simulink subsystem "AeroPropRefFranc"  (R2024b)
settings: Solver=VariableStepAuto  StartTime=0.0  StopTime=10.0  RelTol=1e-3
undefined symbols (not defined in the file or in its folder): ess, Force_b, Fprop_r, geom, H_b, Hdot_b, Moment_b, mot, mot2, mot3, mot4, Mprop_r, propel, propel2, propel3, propel4, pxf_diagram_options, SimIn, SimPar, tc, tc2, tc3, tc4
libraries: simulink x8, slpidlib x4, starslibAxisTransformations x2, libAxisTransformations x2
(part 5 of 10)

== system AeroPropRefFranc/Propulsion and Aerodynamic Forces and Moments/S-Function/Battery Model/powerplant/propel2/plant/parameter_out ==
  inport-propel2_plant_speed_simu : Inport
  inport-propel2_plant_pwr_in_simu : Inport  Port=2
  inport-propel2_plant_pwr_out_simu : Inport  Port=3
  inport-propel2_plant_thrust_simu : Inport  Port=4
  Toworkspace-propel2_plant_pwr_in_simu : ToWorkspace  VariableName=propel2_plant_pwr_in_simu  SampleTime=pxf_diagram_options.workspace_sample_time
      settings: Decimation=pxf_diagram_options.decimation
  Toworkspace-propel2_plant_pwr_out_simu : ToWorkspace  VariableName=propel2_plant_pwr_out_simu  SampleTime=pxf_diagram_options.workspace_sample_time
      settings: Decimation=pxf_diagram_options.decimation
  Toworkspace-propel2_plant_speed_simu : ToWorkspace  VariableName=propel2_plant_speed_simu  SampleTime=pxf_diagram_options.workspace_sample_time
      settings: Decimation=pxf_diagram_options.decimation
  Toworkspace-propel2_plant_thrust_simu : ToWorkspace  VariableName=propel2_plant_thrust_simu  SampleTime=pxf_diagram_options.workspace_sample_time
      settings: Decimation=pxf_diagram_options.decimation
  create_system_info_bus : BusCreator  Inputs=1
  outport-system_info_bus : Outport
  wires:
  inport-propel2_plant_thrust_simu/1 -> Toworkspace-propel2_plant_thrust_simu/1
  inport-propel2_plant_pwr_out_simu/1 -> Toworkspace-propel2_plant_pwr_out_simu/1
  inport-propel2_plant_pwr_in_simu/1 -> Toworkspace-propel2_plant_pwr_in_simu/1
  inport-propel2_plant_speed_simu/1 -> Toworkspace-propel2_plant_speed_simu/1, create_system_info_bus/1  "propel2_plant_speed_simu"
  create_system_info_bus/1 -> outport-system_info_bus/1

== system AeroPropRefFranc/Propulsion and Aerodynamic Forces and Moments/S-Function/Battery Model/powerplant/propel2/plant/parameter_selection ==
  inport-main_info_bus-1 : Inport
  select_main_info_bus : BusSelector  OutputSignals=env_info_bus.env_plant_density_simu,apa_info_bus.powerplant_info_bus.tc.tc_plant_inertia_out_simu,apa_info_bus.apa_plant_info_bus.apa_plant_info_bus.forceeq_bus.eqnmotion_plant_linvel_simu
  outport-env_plant_density_simu-1 : Outport
  outport-tc_plant_inertia_out_simu-2 : Outport  Port=2
  outport-eqnmotion_plant_linvel_simu-3 : Outport  Port=3
  wires:
  select_main_info_bus/3 -> outport-eqnmotion_plant_linvel_simu-3/1  "<eqnmotion_plant_linvel_simu>"
  select_main_info_bus/2 -> outport-tc_plant_inertia_out_simu-2/1  "<tc_plant_inertia_out_simu>"
  select_main_info_bus/1 -> outport-env_plant_density_simu-1/1  "<env_plant_density_simu>"
  inport-main_info_bus-1/1 -> select_main_info_bus/1

== system AeroPropRefFranc/Propulsion and Aerodynamic Forces and Moments/S-Function/Battery Model/powerplant/propel2/plant/propel2_plant_uas ==
  note: rev/s
  note: rad/s
  env_plant_density_simu : Inport
  tc_plant_inertia_out_simu : Inport  Port=2
  eqnmotion_plant_linvel_simu : Inport  Port=3
  tc_plant_trq_out_simu : Inport  Port=4
  flow-in : Inport  Port=5
  Gain : Gain  Gain=propel2.plant.init.thrustdir
  Gain1 : Gain  Gain=2*pi
  Gain2 : Gain
  Gain3 : Gain
  Mux : Mux  Inputs=2
  Propeller Power : Subsystem
  Propeller_CP : Subsystem
  Propeller_Torque : Subsystem
  Terminator : Terminator
  Thrust_Generated : Subsystem
  Total_Moment : Subsystem
  propel_plant_speed_simu : Outport  VectorParamsAs1DForOutWhenUnconnected=off
  propel_plant_pwr_in_simu : Outport  Port=2  VectorParamsAs1DForOutWhenUnconnected=off
  propel_plant_pwr_out_simu : Outport  Port=3  VectorParamsAs1DForOutWhenUnconnected=off
  propel_plant_thrust_simu : Outport  Port=4  VectorParamsAs1DForOutWhenUnconnected=off
  propel_plant_effort : Outport  Port=5  VectorParamsAs1DForOutWhenUnconnected=off
  propel_plant_speed_out_simu : Outport  Port=6  VectorParamsAs1DForOutWhenUnconnected=off
  wires:
  Thrust_Generated/1(propel_plant_thrust_simu) -> propel_plant_thrust_simu/1, Gain/1, Total_Moment/1(propel_plant_thrust_simu), Propeller Power/3(propel_plant_thrust_simu)  "propel_plant_thrust_simu"
  Propeller_Torque/1(propel_plant_rps_simu) -> Thrust_Generated/2(propel_plant_speed_simu), Propeller_CP/1(propel_plant_rps_simu), Gain1/1, Propeller Power/4(propel_plant_rps_simu)
  Propeller_CP/1(propel_plant_CP_simu) -> Propeller_Torque/2(propel_plant_CP_simu), Propeller Power/2(propel_plant_CP_simu)
  Thrust_Generated/2(propel_plant_CT_simu) -> Propeller Power/1(propel_plant_CT_simu)
  env_plant_density_simu/1 -> Propeller_Torque/1(env_plant_density_simu), Thrust_Generated/1(env_plant_density_simu)
  tc_plant_trq_out_simu/1 -> Propeller_Torque/3(tc_plant_trq_out_simu)
  tc_plant_inertia_out_simu/1 -> Propeller_Torque/4(tc_plant_inertia_out_simu)
  Total_Moment/1(accmoment_plant_totmoment_simu) -> Mux/2  "effort_plant_angleffort_simu"
  Propeller_Torque/2(propel_plant_restq_simu) -> Total_Moment/2(propel_plant_restq_simu)
  Gain/1 -> Mux/1  "effort_plant_longeffort_simu"
  Mux/1 -> propel_plant_effort/1  "propel_plant_effort"
  eqnmotion_plant_linvel_simu/1 -> Propeller Power/5(eqnmotion_plant_linvel_simu)
  Gain1/1 -> Gain3/1, Gain2/1
  Propeller Power/2(propel_plant_pwr_out_simu) -> propel_plant_pwr_out_simu/1  "propel_plant_pwr_out_simu"
  Propeller Power/1(propel_plant_pwr_in_simu) -> propel_plant_pwr_in_simu/1  "propel_plant_pwr_in_simu"
  Gain2/1 -> propel_plant_speed_out_simu/1  "propel_plant_speed_out_simu"
  Gain3/1 -> propel_plant_speed_simu/1  "propel_plant_speed_simu"
  flow-in/1 -> Terminator/1

== system AeroPropRefFranc/Propulsion and Aerodynamic Forces and Moments/S-Function/Battery Model/powerplant/propel3/plant/parameter_out ==
  inport-propel3_plant_speed_simu : Inport
  inport-propel3_plant_pwr_in_simu : Inport  Port=2
  inport-propel3_plant_pwr_out_simu : Inport  Port=3
  inport-propel3_plant_thrust_simu : Inport  Port=4
  Toworkspace-propel3_plant_pwr_in_simu : ToWorkspace  VariableName=propel3_plant_pwr_in_simu  SampleTime=pxf_diagram_options.workspace_sample_time
      settings: Decimation=pxf_diagram_options.decimation
  Toworkspace-propel3_plant_pwr_out_simu : ToWorkspace  VariableName=propel3_plant_pwr_out_simu  SampleTime=pxf_diagram_options.workspace_sample_time
      settings: Decimation=pxf_diagram_options.decimation
  Toworkspace-propel3_plant_speed_simu : ToWorkspace  VariableName=propel3_plant_speed_simu  SampleTime=pxf_diagram_options.workspace_sample_time
      settings: Decimation=pxf_diagram_options.decimation
  Toworkspace-propel3_plant_thrust_simu : ToWorkspace  VariableName=propel3_plant_thrust_simu  SampleTime=pxf_diagram_options.workspace_sample_time
      settings: Decimation=pxf_diagram_options.decimation
  create_system_info_bus : BusCreator  Inputs=1
  outport-system_info_bus : Outport
  wires:
  inport-propel3_plant_thrust_simu/1 -> Toworkspace-propel3_plant_thrust_simu/1
  inport-propel3_plant_pwr_out_simu/1 -> Toworkspace-propel3_plant_pwr_out_simu/1
  inport-propel3_plant_pwr_in_simu/1 -> Toworkspace-propel3_plant_pwr_in_simu/1
  inport-propel3_plant_speed_simu/1 -> Toworkspace-propel3_plant_speed_simu/1, create_system_info_bus/1  "propel3_plant_speed_simu"
  create_system_info_bus/1 -> outport-system_info_bus/1

== system AeroPropRefFranc/Propulsion and Aerodynamic Forces and Moments/S-Function/Battery Model/powerplant/propel3/plant/parameter_selection ==
  inport-main_info_bus-1 : Inport
  select_main_info_bus : BusSelector  OutputSignals=env_info_bus.env_plant_density_simu,apa_info_bus.powerplant_info_bus.tc.tc_plant_inertia_out_simu,apa_info_bus.apa_plant_info_bus.apa_plant_info_bus.forceeq_bus.eqnmotion_plant_linvel_simu
  outport-env_plant_density_simu-1 : Outport
  outport-tc_plant_inertia_out_simu-2 : Outport  Port=2
  outport-eqnmotion_plant_linvel_simu-3 : Outport  Port=3
  wires:
  select_main_info_bus/3 -> outport-eqnmotion_plant_linvel_simu-3/1  "<eqnmotion_plant_linvel_simu>"
  select_main_info_bus/2 -> outport-tc_plant_inertia_out_simu-2/1  "<tc_plant_inertia_out_simu>"
  select_main_info_bus/1 -> outport-env_plant_density_simu-1/1  "<env_plant_density_simu>"
  inport-main_info_bus-1/1 -> select_main_info_bus/1

== system AeroPropRefFranc/Propulsion and Aerodynamic Forces and Moments/S-Function/Battery Model/powerplant/propel3/plant/propel3_plant_uas ==
  note: rev/s
  note: rad/s
  env_plant_density_simu : Inport
  tc_plant_inertia_out_simu : Inport  Port=2
  eqnmotion_plant_linvel_simu : Inport  Port=3
  tc_plant_trq_out_simu : Inport  Port=4
  flow-in : Inport  Port=5
  Gain : Gain  Gain=propel3.plant.init.thrustdir
  Gain1 : Gain  Gain=2*pi
  Gain2 : Gain
  Gain3 : Gain
  Mux : Mux  Inputs=2
  Propeller Power : Subsystem
  Propeller_CP : Subsystem
  Propeller_Torque : Subsystem
  Terminator : Terminator
  Thrust_Generated : Subsystem
  Total_Moment : Subsystem
  propel_plant_speed_simu : Outport  VectorParamsAs1DForOutWhenUnconnected=off
  propel_plant_pwr_in_simu : Outport  Port=2  VectorParamsAs1DForOutWhenUnconnected=off
  propel_plant_pwr_out_simu : Outport  Port=3  VectorParamsAs1DForOutWhenUnconnected=off
  propel_plant_thrust_simu : Outport  Port=4  VectorParamsAs1DForOutWhenUnconnected=off
  propel_plant_effort : Outport  Port=5  VectorParamsAs1DForOutWhenUnconnected=off
  propel_plant_speed_out_simu : Outport  Port=6  VectorParamsAs1DForOutWhenUnconnected=off
  wires:
  Thrust_Generated/1(propel_plant_thrust_simu) -> propel_plant_thrust_simu/1, Gain/1, Total_Moment/1(propel_plant_thrust_simu), Propeller Power/3(propel_plant_thrust_simu)  "propel_plant_thrust_simu"
  Propeller_Torque/1(propel_plant_rps_simu) -> Thrust_Generated/2(propel_plant_speed_simu), Propeller_CP/1(propel_plant_rps_simu), Gain1/1, Propeller Power/4(propel_plant_rps_simu)
  Propeller_CP/1(propel_plant_CP_simu) -> Propeller_Torque/2(propel_plant_CP_simu), Propeller Power/2(propel_plant_CP_simu)
  Thrust_Generated/2(propel_plant_CT_simu) -> Propeller Power/1(propel_plant_CT_simu)
  env_plant_density_simu/1 -> Propeller_Torque/1(env_plant_density_simu), Thrust_Generated/1(env_plant_density_simu)
  tc_plant_trq_out_simu/1 -> Propeller_Torque/3(tc_plant_trq_out_simu)
  tc_plant_inertia_out_simu/1 -> Propeller_Torque/4(tc_plant_inertia_out_simu)
  Total_Moment/1(accmoment_plant_totmoment_simu) -> Mux/2  "effort_plant_angleffort_simu"
  Propeller_Torque/2(propel_plant_restq_simu) -> Total_Moment/2(propel_plant_restq_simu)
  Gain/1 -> Mux/1  "effort_plant_longeffort_simu"
  Mux/1 -> propel_plant_effort/1  "propel_plant_effort"
  eqnmotion_plant_linvel_simu/1 -> Propeller Power/5(eqnmotion_plant_linvel_simu)
  Gain1/1 -> Gain3/1, Gain2/1
  Propeller Power/2(propel_plant_pwr_out_simu) -> propel_plant_pwr_out_simu/1  "propel_plant_pwr_out_simu"
  Propeller Power/1(propel_plant_pwr_in_simu) -> propel_plant_pwr_in_simu/1  "propel_plant_pwr_in_simu"
  Gain2/1 -> propel_plant_speed_out_simu/1  "propel_plant_speed_out_simu"
  Gain3/1 -> propel_plant_speed_simu/1  "propel_plant_speed_simu"
  flow-in/1 -> Terminator/1

== system AeroPropRefFranc/Propulsion and Aerodynamic Forces and Moments/S-Function/Battery Model/powerplant/propel4/plant/parameter_out ==
  inport-propel4_plant_speed_simu : Inport
  inport-propel4_plant_pwr_in_simu : Inport  Port=2
  inport-propel4_plant_pwr_out_simu : Inport  Port=3
  inport-propel4_plant_thrust_simu : Inport  Port=4
  Toworkspace-propel4_plant_pwr_in_simu : ToWorkspace  VariableName=propel4_plant_pwr_in_simu  SampleTime=pxf_diagram_options.workspace_sample_time
      settings: Decimation=pxf_diagram_options.decimation
  Toworkspace-propel4_plant_pwr_out_simu : ToWorkspace  VariableName=propel4_plant_pwr_out_simu  SampleTime=pxf_diagram_options.workspace_sample_time
      settings: Decimation=pxf_diagram_options.decimation
  Toworkspace-propel4_plant_speed_simu : ToWorkspace  VariableName=propel4_plant_speed_simu  SampleTime=pxf_diagram_options.workspace_sample_time
      settings: Decimation=pxf_diagram_options.decimation
  Toworkspace-propel4_plant_thrust_simu : ToWorkspace  VariableName=propel4_plant_thrust_simu  SampleTime=pxf_diagram_options.workspace_sample_time
      settings: Decimation=pxf_diagram_options.decimation
  create_system_info_bus : BusCreator  Inputs=1
  outport-system_info_bus : Outport
  wires:
  inport-propel4_plant_thrust_simu/1 -> Toworkspace-propel4_plant_thrust_simu/1
  inport-propel4_plant_pwr_out_simu/1 -> Toworkspace-propel4_plant_pwr_out_simu/1
  inport-propel4_plant_pwr_in_simu/1 -> Toworkspace-propel4_plant_pwr_in_simu/1
  inport-propel4_plant_speed_simu/1 -> Toworkspace-propel4_plant_speed_simu/1, create_system_info_bus/1  "propel4_plant_speed_simu"
  create_system_info_bus/1 -> outport-system_info_bus/1

== system AeroPropRefFranc/Propulsion and Aerodynamic Forces and Moments/S-Function/Battery Model/powerplant/propel4/plant/parameter_selection ==
  inport-main_info_bus-1 : Inport
  select_main_info_bus : BusSelector  OutputSignals=env_info_bus.env_plant_density_simu,apa_info_bus.powerplant_info_bus.tc.tc_plant_inertia_out_simu,apa_info_bus.apa_plant_info_bus.apa_plant_info_bus.forceeq_bus.eqnmotion_plant_linvel_simu
  outport-env_plant_density_simu-1 : Outport
  outport-tc_plant_inertia_out_simu-2 : Outport  Port=2
  outport-eqnmotion_plant_linvel_simu-3 : Outport  Port=3
  wires:
  select_main_info_bus/3 -> outport-eqnmotion_plant_linvel_simu-3/1  "<eqnmotion_plant_linvel_simu>"
  select_main_info_bus/2 -> outport-tc_plant_inertia_out_simu-2/1  "<tc_plant_inertia_out_simu>"
  select_main_info_bus/1 -> outport-env_plant_density_simu-1/1  "<env_plant_density_simu>"
  inport-main_info_bus-1/1 -> select_main_info_bus/1

== system AeroPropRefFranc/Propulsion and Aerodynamic Forces and Moments/S-Function/Battery Model/powerplant/propel4/plant/propel4_plant_uas ==
  note: rev/s
  note: rad/s
  env_plant_density_simu : Inport
  tc_plant_inertia_out_simu : Inport  Port=2
  eqnmotion_plant_linvel_simu : Inport  Port=3
  tc_plant_trq_out_simu : Inport  Port=4
  flow-in : Inport  Port=5
  Gain : Gain  Gain=propel4.plant.init.thrustdir
  Gain1 : Gain  Gain=2*pi
  Gain2 : Gain
  Gain3 : Gain
  Mux : Mux  Inputs=2
  Propeller Power : Subsystem
  Propeller_CP : Subsystem
  Propeller_Torque : Subsystem
  Terminator : Terminator
  Thrust_Generated : Subsystem
  Total_Moment : Subsystem
  propel_plant_speed_simu : Outport  VectorParamsAs1DForOutWhenUnconnected=off
  propel_plant_pwr_in_simu : Outport  Port=2  VectorParamsAs1DForOutWhenUnconnected=off
  propel_plant_pwr_out_simu : Outport  Port=3  VectorParamsAs1DForOutWhenUnconnected=off
  propel_plant_thrust_simu : Outport  Port=4  VectorParamsAs1DForOutWhenUnconnected=off
  propel_plant_effort : Outport  Port=5  VectorParamsAs1DForOutWhenUnconnected=off
  propel_plant_speed_out_simu : Outport  Port=6  VectorParamsAs1DForOutWhenUnconnected=off
  wires:
  Thrust_Generated/1(propel_plant_thrust_simu) -> propel_plant_thrust_simu/1, Gain/1, Total_Moment/1(propel_plant_thrust_simu), Propeller Power/3(propel_plant_thrust_simu)  "propel_plant_thrust_simu"
  Propeller_Torque/1(propel_plant_rps_simu) -> Thrust_Generated/2(propel_plant_speed_simu), Propeller_CP/1(propel_plant_rps_simu), Gain1/1, Propeller Power/4(propel_plant_rps_simu)
  Propeller_CP/1(propel_plant_CP_simu) -> Propeller_Torque/2(propel_plant_CP_simu), Propeller Power/2(propel_plant_CP_simu)
  Thrust_Generated/2(propel_plant_CT_simu) -> Propeller Power/1(propel_plant_CT_simu)
  env_plant_density_simu/1 -> Propeller_Torque/1(env_plant_density_simu), Thrust_Generated/1(env_plant_density_simu)
  tc_plant_trq_out_simu/1 -> Propeller_Torque/3(tc_plant_trq_out_simu)
  tc_plant_inertia_out_simu/1 -> Propeller_Torque/4(tc_plant_inertia_out_simu)
  Total_Moment/1(accmoment_plant_totmoment_simu) -> Mux/2  "effort_plant_angleffort_simu"
  Propeller_Torque/2(propel_plant_restq_simu) -> Total_Moment/2(propel_plant_restq_simu)
  Gain/1 -> Mux/1  "effort_plant_longeffort_simu"
  Mux/1 -> propel_plant_effort/1  "propel_plant_effort"
  eqnmotion_plant_linvel_simu/1 -> Propeller Power/5(eqnmotion_plant_linvel_simu)
  Gain1/1 -> Gain3/1, Gain2/1
  Propeller Power/2(propel_plant_pwr_out_simu) -> propel_plant_pwr_out_simu/1  "propel_plant_pwr_out_simu"
  Propeller Power/1(propel_plant_pwr_in_simu) -> propel_plant_pwr_in_simu/1  "propel_plant_pwr_in_simu"
  Gain2/1 -> propel_plant_speed_out_simu/1  "propel_plant_speed_out_simu"
  Gain3/1 -> propel_plant_speed_simu/1  "propel_plant_speed_simu"
  flow-in/1 -> Terminator/1

== system AeroPropRefFranc/Propulsion and Aerodynamic Forces and Moments/S-Function/Battery Model/powerplant/tc/plant/parameter_out ==
  inport-tc_plant_trq_in_simu : Inport
  inport-tc_plant_trq_out_simu : Inport  Port=2
  inport-tc_plant_spd_in_simu : Inport  Port=3
  inport-tc_plant_spd_out_simu : Inport  Port=4
  inport-tc_plant_inertia_in_simu : Inport  Port=5
  inport-tc_plant_inertia_out_simu : Inport  Port=6
  Toworkspace-tc_plant_inertia_in_simu : ToWorkspace  VariableName=tc_plant_inertia_in_simu  SampleTime=pxf_diagram_options.workspace_sample_time
      settings: Decimation=pxf_diagram_options.decimation
  Toworkspace-tc_plant_inertia_out_simu : ToWorkspace  VariableName=tc_plant_inertia_out_simu  SampleTime=pxf_diagram_options.workspace_sample_time
      settings: Decimation=pxf_diagram_options.decimation
  Toworkspace-tc_plant_spd_in_simu : ToWorkspace  VariableName=tc_plant_spd_in_simu  SampleTime=pxf_diagram_options.workspace_sample_time
      settings: Decimation=pxf_diagram_options.decimation
  Toworkspace-tc_plant_spd_out_simu : ToWorkspace  VariableName=tc_plant_spd_out_simu  SampleTime=pxf_diagram_options.workspace_sample_time
      settings: Decimation=pxf_diagram_options.decimation
  Toworkspace-tc_plant_trq_in_simu : ToWorkspace  VariableName=tc_plant_trq_in_simu  SampleTime=pxf_diagram_options.workspace_sample_time
      settings: Decimation=pxf_diagram_options.decimation
  Toworkspace-tc_plant_trq_out_simu : ToWorkspace  VariableName=tc_plant_trq_out_simu  SampleTime=pxf_diagram_options.workspace_sample_time
      settings: Decimation=pxf_diagram_options.decimation
  create_system_info_bus : BusCreator  Inputs=2
  outport-system_info_bus : Outport
  wires:
  inport-tc_plant_inertia_out_simu/1 -> Toworkspace-tc_plant_inertia_out_simu/1, create_system_info_bus/2  "tc_plant_inertia_out_simu"
  inport-tc_plant_inertia_in_simu/1 -> Toworkspace-tc_plant_inertia_in_simu/1
  inport-tc_plant_spd_out_simu/1 -> Toworkspace-tc_plant_spd_out_simu/1
  inport-tc_plant_spd_in_simu/1 -> Toworkspace-tc_plant_spd_in_simu/1, create_system_info_bus/1  "tc_plant_spd_in_simu"
  inport-tc_plant_trq_out_simu/1 -> Toworkspace-tc_plant_trq_out_simu/1
  inport-tc_plant_trq_in_simu/1 -> Toworkspace-tc_plant_trq_in_simu/1
  create_system_info_bus/1 -> outport-system_info_bus/1

== system AeroPropRefFranc/Propulsion and Aerodynamic Forces and Moments/S-Function/Battery Model/powerplant/tc/plant/parameter_selection ==

== system AeroPropRefFranc/Propulsion and Aerodynamic Forces and Moments/S-Function/Battery Model/powerplant/tc/plant/tc_plant_map_trqloss_funTW ==
  tc_trq_in tc_inertia_in : Inport
  tc_spd_out : Inport  Port=2
  Demux : Demux  Outputs=2
  Inertia calculation : Subsystem
  Mux1 : Mux  Inputs=2
  Speed calculation : Subsystem
  Torque calculation : Subsystem
  tc_plant_trq_in_simu : Outport
  tc_plant_trq_out_simu : Outport  Port=2
  tc_plant_spd_in_simu : Outport  Port=3
  tc_plant_spd_out_simu : Outport  Port=4
  tc_plant_inertia_in_simu : Outport  Port=5
  tc_plant_inertia_out_simu : Outport  Port=6
  tc_trq_out : Outport  Port=7
  tc_spd_in : Outport  Port=8
  wires:
  Speed calculation/1(spd in) -> tc_spd_in/1, [tc_plant_spd_in_simu], Torque calculation/1(spd in)
  tc_spd_out/1 -> Speed calculation/1(spd out), [tc_plant_spd_out_simu]
  Demux/1 -> [tc_plant_trq_in_simu], Torque calculation/2(trq in)
  Demux/2 -> Inertia calculation/1(inertia in), [tc_plant_inertia_in_simu]
  Inertia calculation/1(inertia out) -> Mux1/2, [tc_plant_inertia_out_simu]  "tc_plant_inertia_out_simu"
  Torque calculation/1(trq out) -> Mux1/1, [tc_plant_trq_out_simu]  "tc_plant_trq_out_simu"
  [tc_plant_inertia_out_simu] -> tc_plant_inertia_out_simu/1  "tc_plant_inertia_out_simu"
  [tc_plant_inertia_in_simu] -> tc_plant_inertia_in_simu/1  "tc_plant_inertia_in_simu"
  [tc_plant_spd_out_simu] -> tc_plant_spd_out_simu/1  "tc_plant_spd_out_simu"
  [tc_plant_spd_in_simu] -> tc_plant_spd_in_simu/1  "tc_plant_spd_in_simu"
  [tc_plant_trq_out_simu] -> tc_plant_trq_out_simu/1  "tc_plant_trq_out_simu"
  [tc_plant_trq_in_simu] -> tc_plant_trq_in_simu/1  "tc_plant_trq_in_simu"
  Mux1/1 -> tc_trq_out/1
  tc_trq_in tc_inertia_in/1 -> Demux/1

== system AeroPropRefFranc/Propulsion and Aerodynamic Forces and Moments/S-Function/Battery Model/powerplant/tc2/plant/parameter_out ==
  inport-tc2_plant_trq_in_simu : Inport
  inport-tc2_plant_trq_out_simu : Inport  Port=2
  inport-tc2_plant_spd_in_simu : Inport  Port=3
  inport-tc2_plant_spd_out_simu : Inport  Port=4
  inport-tc2_plant_inertia_in_simu : Inport  Port=5
  inport-tc2_plant_inertia_out_simu : Inport  Port=6
  Toworkspace-tc2_plant_inertia_in_simu : ToWorkspace  VariableName=tc2_plant_inertia_in_simu  SampleTime=pxf_diagram_options.workspace_sample_time
      settings: Decimation=pxf_diagram_options.decimation
  Toworkspace-tc2_plant_inertia_out_simu : ToWorkspace  VariableName=tc2_plant_inertia_out_simu  SampleTime=pxf_diagram_options.workspace_sample_time
      settings: Decimation=pxf_diagram_options.decimation
  Toworkspace-tc2_plant_spd_in_simu : ToWorkspace  VariableName=tc2_plant_spd_in_simu  SampleTime=pxf_diagram_options.workspace_sample_time
      settings: Decimation=pxf_diagram_options.decimation
  Toworkspace-tc2_plant_spd_out_simu : ToWorkspace  VariableName=tc2_plant_spd_out_simu  SampleTime=pxf_diagram_options.workspace_sample_time
      settings: Decimation=pxf_diagram_options.decimation
  Toworkspace-tc2_plant_trq_in_simu : ToWorkspace  VariableName=tc2_plant_trq_in_simu  SampleTime=pxf_diagram_options.workspace_sample_time
      settings: Decimation=pxf_diagram_options.decimation
  Toworkspace-tc2_plant_trq_out_simu : ToWorkspace  VariableName=tc2_plant_trq_out_simu  SampleTime=pxf_diagram_options.workspace_sample_time
      settings: Decimation=pxf_diagram_options.decimation
  create_system_info_bus : BusCreator  Inputs=1
  outport-system_info_bus : Outport
  wires:
  inport-tc2_plant_inertia_out_simu/1 -> Toworkspace-tc2_plant_inertia_out_simu/1
  inport-tc2_plant_inertia_in_simu/1 -> Toworkspace-tc2_plant_inertia_in_simu/1
  inport-tc2_plant_spd_out_simu/1 -> Toworkspace-tc2_plant_spd_out_simu/1
  inport-tc2_plant_spd_in_simu/1 -> Toworkspace-tc2_plant_spd_in_simu/1, create_system_info_bus/1  "tc2_plant_spd_in_simu"
  inport-tc2_plant_trq_out_simu/1 -> Toworkspace-tc2_plant_trq_out_simu/1
  inport-tc2_plant_trq_in_simu/1 -> Toworkspace-tc2_plant_trq_in_simu/1
  create_system_info_bus/1 -> outport-system_info_bus/1

== system AeroPropRefFranc/Propulsion and Aerodynamic Forces and Moments/S-Function/Battery Model/powerplant/tc2/plant/parameter_selection ==

== system AeroPropRefFranc/Propulsion and Aerodynamic Forces and Moments/S-Function/Battery Model/powerplant/tc2/plant/tc2_plant_map_trqloss_funTW ==
  tc_trq_in tc_inertia_in : Inport
  tc_spd_out : Inport  Port=2
  Demux : Demux  Outputs=2
  Inertia calculation : Subsystem
  Mux1 : Mux  Inputs=2
  Speed calculation : Subsystem
  Torque calculation : Subsystem
  tc_plant_trq_in_simu : Outport
  tc_plant_trq_out_simu : Outport  Port=2
  tc_plant_spd_in_simu : Outport  Port=3
  tc_plant_spd_out_simu : Outport  Port=4
  tc_plant_inertia_in_simu : Outport  Port=5
  tc_plant_inertia_out_simu : Outport  Port=6
  tc_trq_out : Outport  Port=7
  tc_spd_in : Outport  Port=8
  wires:
  Speed calculation/1(spd in) -> tc_spd_in/1, [tc2_plant_spd_in_simu], Torque calculation/1(spd in)
  tc_spd_out/1 -> Speed calculation/1(spd out), [tc2_plant_spd_out_simu]
  Demux/1 -> [tc2_plant_trq_in_simu], Torque calculation/2(trq in)
  Demux/2 -> Inertia calculation/1(inertia in), [tc2_plant_inertia_in_simu]
  Inertia calculation/1(inertia out) -> Mux1/2, [tc2_plant_inertia_out_simu]  "tc_plant_inertia_out_simu"
  Torque calculation/1(trq out) -> Mux1/1, [tc2_plant_trq_out_simu]  "tc_plant_trq_out_simu"
  [tc2_plant_inertia_out_simu] -> tc_plant_inertia_out_simu/1  "tc_plant_inertia_out_simu"
  [tc2_plant_inertia_in_simu] -> tc_plant_inertia_in_simu/1  "tc_plant_inertia_in_simu"
  [tc2_plant_spd_out_simu] -> tc_plant_spd_out_simu/1  "tc_plant_spd_out_simu"
  [tc2_plant_spd_in_simu] -> tc_plant_spd_in_simu/1  "tc_plant_spd_in_simu"
  [tc2_plant_trq_out_simu] -> tc_plant_trq_out_simu/1  "tc_plant_trq_out_simu"
  [tc2_plant_trq_in_simu] -> tc_plant_trq_in_simu/1  "tc_plant_trq_in_simu"
  Mux1/1 -> tc_trq_out/1
  tc_trq_in tc_inertia_in/1 -> Demux/1

== system AeroPropRefFranc/Propulsion and Aerodynamic Forces and Moments/S-Function/Battery Model/powerplant/tc3/plant/parameter_out ==
  inport-tc3_plant_trq_in_simu : Inport
  inport-tc3_plant_trq_out_simu : Inport  Port=2
  inport-tc3_plant_spd_in_simu : Inport  Port=3
  inport-tc3_plant_spd_out_simu : Inport  Port=4
  inport-tc3_plant_inertia_in_simu : Inport  Port=5
  inport-tc3_plant_inertia_out_simu : Inport  Port=6
  Toworkspace-tc3_plant_inertia_in_simu : ToWorkspace  VariableName=tc3_plant_inertia_in_simu  SampleTime=pxf_diagram_options.workspace_sample_time
      settings: Decimation=pxf_diagram_options.decimation
  Toworkspace-tc3_plant_inertia_out_simu : ToWorkspace  VariableName=tc3_plant_inertia_out_simu  SampleTime=pxf_diagram_options.workspace_sample_time
      settings: Decimation=pxf_diagram_options.decimation
  Toworkspace-tc3_plant_spd_in_simu : ToWorkspace  VariableName=tc3_plant_spd_in_simu  SampleTime=pxf_diagram_options.workspace_sample_time
      settings: Decimation=pxf_diagram_options.decimation
  Toworkspace-tc3_plant_spd_out_simu : ToWorkspace  VariableName=tc3_plant_spd_out_simu  SampleTime=pxf_diagram_options.workspace_sample_time
      settings: Decimation=pxf_diagram_options.decimation
  Toworkspace-tc3_plant_trq_in_simu : ToWorkspace  VariableName=tc3_plant_trq_in_simu  SampleTime=pxf_diagram_options.workspace_sample_time
      settings: Decimation=pxf_diagram_options.decimation
  Toworkspace-tc3_plant_trq_out_simu : ToWorkspace  VariableName=tc3_plant_trq_out_simu  SampleTime=pxf_diagram_options.workspace_sample_time
      settings: Decimation=pxf_diagram_options.decimation
  create_system_info_bus : BusCreator  Inputs=1
  outport-system_info_bus : Outport
  wires:
  inport-tc3_plant_inertia_out_simu/1 -> Toworkspace-tc3_plant_inertia_out_simu/1
  inport-tc3_plant_inertia_in_simu/1 -> Toworkspace-tc3_plant_inertia_in_simu/1
  inport-tc3_plant_spd_out_simu/1 -> Toworkspace-tc3_plant_spd_out_simu/1
  inport-tc3_plant_spd_in_simu/1 -> Toworkspace-tc3_plant_spd_in_simu/1, create_system_info_bus/1  "tc3_plant_spd_in_simu"
  inport-tc3_plant_trq_out_simu/1 -> Toworkspace-tc3_plant_trq_out_simu/1
  inport-tc3_plant_trq_in_simu/1 -> Toworkspace-tc3_plant_trq_in_simu/1
  create_system_info_bus/1 -> outport-system_info_bus/1

== system AeroPropRefFranc/Propulsion and Aerodynamic Forces and Moments/S-Function/Battery Model/powerplant/tc3/plant/parameter_selection ==

== system AeroPropRefFranc/Propulsion and Aerodynamic Forces and Moments/S-Function/Battery Model/powerplant/tc3/plant/tc3_plant_map_trqloss_funTW ==
  tc_trq_in tc_inertia_in : Inport
  tc_spd_out : Inport  Port=2
  Demux : Demux  Outputs=2
  Inertia calculation : Subsystem
  Mux1 : Mux  Inputs=2
  Speed calculation : Subsystem
  Torque calculation : Subsystem
  tc_plant_trq_in_simu : Outport
  tc_plant_trq_out_simu : Outport  Port=2
  tc_plant_spd_in_simu : Outport  Port=3
  tc_plant_spd_out_simu : Outport  Port=4
  tc_plant_inertia_in_simu : Outport  Port=5
  tc_plant_inertia_out_simu : Outport  Port=6
  tc_trq_out : Outport  Port=7
  tc_spd_in : Outport  Port=8
  wires:
  Speed calculation/1(spd in) -> tc_spd_in/1, [tc3_plant_spd_in_simu], Torque calculation/1(spd in)
  tc_spd_out/1 -> Speed calculation/1(spd out), [tc3_plant_spd_out_simu]
  Demux/1 -> [tc3_plant_trq_in_simu], Torque calculation/2(trq in)
  Demux/2 -> Inertia calculation/1(inertia in), [tc3_plant_inertia_in_simu]
  Inertia calculation/1(inertia out) -> Mux1/2, [tc3_plant_inertia_out_simu]  "tc_plant_inertia_out_simu"
  Torque calculation/1(trq out) -> Mux1/1, [tc3_plant_trq_out_simu]  "tc_plant_trq_out_simu"
  [tc3_plant_inertia_out_simu] -> tc_plant_inertia_out_simu/1  "tc_plant_inertia_out_simu"
  [tc3_plant_inertia_in_simu] -> tc_plant_inertia_in_simu/1  "tc_plant_inertia_in_simu"
  [tc3_plant_spd_out_simu] -> tc_plant_spd_out_simu/1  "tc_plant_spd_out_simu"
  [tc3_plant_spd_in_simu] -> tc_plant_spd_in_simu/1  "tc_plant_spd_in_simu"
  [tc3_plant_trq_out_simu] -> tc_plant_trq_out_simu/1  "tc_plant_trq_out_simu"
  [tc3_plant_trq_in_simu] -> tc_plant_trq_in_simu/1  "tc_plant_trq_in_simu"
  Mux1/1 -> tc_trq_out/1
  tc_trq_in tc_inertia_in/1 -> Demux/1

== system AeroPropRefFranc/Propulsion and Aerodynamic Forces and Moments/S-Function/Battery Model/powerplant/tc4/plant/parameter_out ==
  inport-tc4_plant_trq_in_simu : Inport
  inport-tc4_plant_trq_out_simu : Inport  Port=2
  inport-tc4_plant_spd_in_simu : Inport  Port=3
  inport-tc4_plant_spd_out_simu : Inport  Port=4
  inport-tc4_plant_inertia_in_simu : Inport  Port=5
  inport-tc4_plant_inertia_out_simu : Inport  Port=6
  Toworkspace-tc4_plant_inertia_in_simu : ToWorkspace  VariableName=tc4_plant_inertia_in_simu  SampleTime=pxf_diagram_options.workspace_sample_time
      settings: Decimation=pxf_diagram_options.decimation
  Toworkspace-tc4_plant_inertia_out_simu : ToWorkspace  VariableName=tc4_plant_inertia_out_simu  SampleTime=pxf_diagram_options.workspace_sample_time
      settings: Decimation=pxf_diagram_options.decimation
  Toworkspace-tc4_plant_spd_in_simu : ToWorkspace  VariableName=tc4_plant_spd_in_simu  SampleTime=pxf_diagram_options.workspace_sample_time
      settings: Decimation=pxf_diagram_options.decimation
  Toworkspace-tc4_plant_spd_out_simu : ToWorkspace  VariableName=tc4_plant_spd_out_simu  SampleTime=pxf_diagram_options.workspace_sample_time
      settings: Decimation=pxf_diagram_options.decimation
  Toworkspace-tc4_plant_trq_in_simu : ToWorkspace  VariableName=tc4_plant_trq_in_simu  SampleTime=pxf_diagram_options.workspace_sample_time
      settings: Decimation=pxf_diagram_options.decimation
  Toworkspace-tc4_plant_trq_out_simu : ToWorkspace  VariableName=tc4_plant_trq_out_simu  SampleTime=pxf_diagram_options.workspace_sample_time
      settings: Decimation=pxf_diagram_options.decimation
  create_system_info_bus : BusCreator  Inputs=1
  outport-system_info_bus : Outport
  wires:
  inport-tc4_plant_inertia_out_simu/1 -> Toworkspace-tc4_plant_inertia_out_simu/1
  inport-tc4_plant_inertia_in_simu/1 -> Toworkspace-tc4_plant_inertia_in_simu/1
  inport-tc4_plant_spd_out_simu/1 -> Toworkspace-tc4_plant_spd_out_simu/1
  inport-tc4_plant_spd_in_simu/1 -> Toworkspace-tc4_plant_spd_in_simu/1, create_system_info_bus/1  "tc4_plant_spd_in_simu"
  inport-tc4_plant_trq_out_simu/1 -> Toworkspace-tc4_plant_trq_out_simu/1
  inport-tc4_plant_trq_in_simu/1 -> Toworkspace-tc4_plant_trq_in_simu/1
  create_system_info_bus/1 -> outport-system_info_bus/1

== system AeroPropRefFranc/Propulsion and Aerodynamic Forces and Moments/S-Function/Battery Model/powerplant/tc4/plant/parameter_selection ==

== system AeroPropRefFranc/Propulsion and Aerodynamic Forces and Moments/S-Function/Battery Model/powerplant/tc4/plant/tc4_plant_map_trqloss_funTW ==
  tc_trq_in tc_inertia_in : Inport
  tc_spd_out : Inport  Port=2
  Demux : Demux  Outputs=2
  Inertia calculation : Subsystem
  Mux1 : Mux  Inputs=2
  Speed calculation : Subsystem
  Torque calculation : Subsystem
  tc_plant_trq_in_simu : Outport
  tc_plant_trq_out_simu : Outport  Port=2
  tc_plant_spd_in_simu : Outport  Port=3
  tc_plant_spd_out_simu : Outport  Port=4
  tc_plant_inertia_in_simu : Outport  Port=5
  tc_plant_inertia_out_simu : Outport  Port=6
  tc_trq_out : Outport  Port=7
  tc_spd_in : Outport  Port=8
  wires:
  Speed calculation/1(spd in) -> tc_spd_in/1, [tc4_plant_spd_in_simu], Torque calculation/1(spd in)
  tc_spd_out/1 -> Speed calculation/1(spd out), [tc4_plant_spd_out_simu]
  Demux/1 -> [tc4_plant_trq_in_simu], Torque calculation/2(trq in)
  Demux/2 -> Inertia calculation/1(inertia in), [tc4_plant_inertia_in_simu]
  Inertia calculation/1(inertia out) -> Mux1/2, [tc4_plant_inertia_out_simu]  "tc_plant_inertia_out_simu"
  Torque calculation/1(trq out) -> Mux1/1, [tc4_plant_trq_out_simu]  "tc_plant_trq_out_simu"
  [tc4_plant_inertia_out_simu] -> tc_plant_inertia_out_simu/1  "tc_plant_inertia_out_simu"
  [tc4_plant_inertia_in_simu] -> tc_plant_inertia_in_simu/1  "tc_plant_inertia_in_simu"
  [tc4_plant_spd_out_simu] -> tc_plant_spd_out_simu/1  "tc_plant_spd_out_simu"
  [tc4_plant_spd_in_simu] -> tc_plant_spd_in_simu/1  "tc_plant_spd_in_simu"
  [tc4_plant_trq_out_simu] -> tc_plant_trq_out_simu/1  "tc_plant_trq_out_simu"
  [tc4_plant_trq_in_simu] -> tc_plant_trq_in_simu/1  "tc_plant_trq_in_simu"
  Mux1/1 -> tc_trq_out/1
  tc_trq_in tc_inertia_in/1 -> Demux/1

== system AeroPropRefFranc/Propulsion and Aerodynamic Forces and Moments/S-Function/Battery Model/ess (battery)/ctrl/ess_ctrl_pngv_map_anl_PI_cstr/PI controller for maximal charge power and current1/PI Ratio Calculator (curr)  ==
  note: %deviation
  ess curr : Inport
  curr max cont : Inport  Port=2
  Add1 : Sum  Inputs=-+
  Integrator1 : Integrator  InitialCondition=ess.plant.init.ul_curr_chg  LimitOutput=on  UpperSaturationLimit=ess.plant.init.ul_curr_chg  LowerSaturationLimit=ess.plant.init.ll_curr_chg
  Ki_curr : Gain  Gain=ess.plant.init.Ki_curr_chg  SaturateOnIntegerOverflow=on  OutDataTypeStr=Inherit: Same as input  ParamDataTypeStr=Inherit: Same as input
  Saturation1 : Saturate  UpperLimit=1  LowerLimit=0
  non-zero division1 : Subsystem
      mask Display: disp('divider')
  Current ratio : Outport
  wires:
  curr max cont/1 -> non-zero division1/2(In2), Add1/2
  Saturation1/1 -> Current ratio/1
  ess curr/1 -> Add1/1
  Integrator1/1 -> Saturation1/1
  Ki_curr/1 -> Integrator1/1
  non-zero division1/1(Out1) -> Ki_curr/1
  Add1/1 -> non-zero division1/1(In1)

== system AeroPropRefFranc/Propulsion and Aerodynamic Forces and Moments/S-Function/Battery Model/ess (battery)/ctrl/ess_ctrl_pngv_map_anl_PI_cstr/PI controller for maximal charge power and current1/PI Ratio Calculator (curr) 1 ==
  note: %deviation
  ess pwr : Inport
  pwr max cont : Inport  Port=2
  Add1 : Sum  Inputs=-+
  Integrator1 : Integrator  InitialCondition=ess.plant.init.ul_curr_dis  LimitOutput=on  UpperSaturationLimit=ess.plant.init.ul_curr_dis  LowerSaturationLimit=ess.plant.init.ll_curr_dis
  Ki_pwr : Gain  Gain=ess.plant.init.Ki_pwr_chg  SaturateOnIntegerOverflow=on  OutDataTypeStr=Inherit: Same as input  ParamDataTypeStr=Inherit: Same as input
  Saturation1 : Saturate  UpperLimit=1  LowerLimit=0
  non-zero division1 : Subsystem
      mask Display: disp('divider')
  pwr ratio : Outport
  wires:
  pwr max cont/1 -> non-zero division1/2(In2), Add1/2
  Saturation1/1 -> pwr ratio/1
  ess pwr/1 -> Add1/1
  Integrator1/1 -> Saturation1/1
  Ki_pwr/1 -> Integrator1/1
  non-zero division1/1(Out1) -> Ki_pwr/1
  Add1/1 -> non-zero division1/1(In1)

== system AeroPropRefFranc/Propulsion and Aerodynamic Forces and Moments/S-Function/Battery Model/ess (battery)/ctrl/ess_ctrl_pngv_map_anl_PI_cstr/PI controller for maximal discharge power and current1/PI Ratio Calculator (curr)  ==
  note: %deviation
  ess curr : Inport
  curr max cont : Inport  Port=2
  Add1 : Sum  Inputs=-+
  Integrator1 : Integrator  InitialCondition=ess.plant.init.ul_curr_dis  LimitOutput=on  UpperSaturationLimit=ess.plant.init.ul_curr_dis  LowerSaturationLimit=ess.plant.init.ll_curr_dis
  Ki_curr : Gain  Gain=ess.plant.init.Ki_curr_dis  SaturateOnIntegerOverflow=on  OutDataTypeStr=Inherit: Same as input  ParamDataTypeStr=Inherit: Same as input
  Saturation1 : Saturate  UpperLimit=1  LowerLimit=0
  non-zero division1 : Subsystem
      mask Display: disp('divider')
  Current ratio : Outport
  wires:
  Add1/1 -> non-zero division1/1(In1)
  non-zero division1/1(Out1) -> Ki_curr/1
  Ki_curr/1 -> Integrator1/1
  Integrator1/1 -> Saturation1/1
  ess curr/1 -> Add1/1
  Saturation1/1 -> Current ratio/1
  curr max cont/1 -> Add1/2, non-zero division1/2(In2)

== system AeroPropRefFranc/Propulsion and Aerodynamic Forces and Moments/S-Function/Battery Model/ess (battery)/ctrl/ess_ctrl_pngv_map_anl_PI_cstr/PI controller for maximal discharge power and current1/PI Ratio Calculator (curr) 1 ==
  note: %deviation
  ess pwr : Inport
  pwr max cont : Inport  Port=2
  Add1 : Sum  Inputs=-+
  Integrator1 : Integrator  InitialCondition=ess.plant.init.ul_curr_dis  LimitOutput=on  UpperSaturationLimit=ess.plant.init.ul_curr_dis  LowerSaturationLimit=ess.plant.init.ll_curr_dis
  Ki_pwr : Gain  Gain=ess.plant.init.Ki_pwr_dis  SaturateOnIntegerOverflow=on  OutDataTypeStr=Inherit: Same as input  ParamDataTypeStr=Inherit: Same as input
  Saturation1 : Saturate  UpperLimit=1  LowerLimit=0
  non-zero division1 : Subsystem
      mask Display: disp('divider')
  pwr ratio : Outport
  wires:
  pwr max cont/1 -> non-zero division1/2(In2), Add1/2
  Saturation1/1 -> pwr ratio/1
  ess pwr/1 -> Add1/1
  Integrator1/1 -> Saturation1/1
  Ki_pwr/1 -> Integrator1/1
  non-zero division1/1(Out1) -> Ki_pwr/1
  Add1/1 -> non-zero division1/1(In1)

== system AeroPropRefFranc/Propulsion and Aerodynamic Forces and Moments/S-Function/Battery Model/ess (battery)/plant/ess_plant_pngv_map_anl_PI_cstr/ess_cell/current polarization ==
  ess soc : Inport
  ess curr : Inport  Port=2
  Integrator : Integrator
  Product1 : Product  Inputs=*/  InputSameDT=on  SaturateOnIntegerOverflow=on  OutDataTypeStr=Inherit: Same as first input
  Sum1 : Sum  Inputs=+-  InputSameDT=on  SaturateOnIntegerOverflow=on  OutDataTypeStr=Inherit: Same as first input
  Time Constant : Lookup  InputValues=ess.plant.init.tau1.idx1_soc  Table=ess.plant.init.tau1.map
  ess_cell_curr_polar1 : Outport
  wires:
  Integrator/1 -> ess_cell_curr_polar1/1, Sum1/2
  Sum1/1 -> Product1/1
  ess curr/1 -> Sum1/1
  ess soc/1 -> Time Constant/1
  Product1/1 -> Integrator/1
  Time Constant/1 -> Product1/2

== system AeroPropRefFranc/Propulsion and Aerodynamic Forces and Moments/S-Function/Battery Model/ess (battery)/plant/ess_plant_pngv_map_anl_PI_cstr/ess_cell/current polarization1 ==
  ess soc : Inport
  ess curr : Inport  Port=2
  Integrator : Integrator
  Product1 : Product  Inputs=*/  InputSameDT=on  SaturateOnIntegerOverflow=on  OutDataTypeStr=Inherit: Same as first input
  Sum1 : Sum  Inputs=+-  InputSameDT=on  SaturateOnIntegerOverflow=on  OutDataTypeStr=Inherit: Same as first input
  Time Constant : Lookup  InputValues=ess.plant.init.tau2.idx1_soc  Table=ess.plant.init.tau2.map
  ess_cell_curr_polar2 : Outport
  wires:
  Time Constant/1 -> Product1/2
  Product1/1 -> Integrator/1
  ess soc/1 -> Time Constant/1
  ess curr/1 -> Sum1/1
  Sum1/1 -> Product1/1
  Integrator/1 -> Sum1/2, ess_cell_curr_polar2/1

== system AeroPropRefFranc/Propulsion and Aerodynamic Forces and Moments/S-Function/Battery Model/ess (battery)/plant/ess_plant_pngv_map_anl_PI_cstr/ess_cell/ess_soc_calculation ==
  cell_curr : Inport
  (sec->hrs) : Gain  Gain=1/3600  SaturateOnIntegerOverflow=on  OutDataTypeStr=Inherit: Same as input  ParamDataTypeStr=Inherit: Same as input
  (sec->hrs)1 : Gain  Gain=-1  SaturateOnIntegerOverflow=on  OutDataTypeStr=Inherit: Same as input  ParamDataTypeStr=Inherit: Same as input
  0 <= SOC <= 1 : Saturate  UpperLimit=1  LowerLimit=0
  1\ess.plant.init.cap : Gain  Gain=1/ess.plant.init.cap  SaturateOnIntegerOverflow=on  OutDataTypeStr=Inherit: Same as input  ParamDataTypeStr=Inherit: Same as input
  Integrator : Integrator  InitialCondition=ess.plant.init.soc_init
  ess_soc : Outport
  wires:
  cell_curr/1 -> (sec->hrs)/1
  1\ess.plant.init.cap/1 -> (sec->hrs)1/1
  (sec->hrs)1/1 -> Integrator/1
  Integrator/1 -> 0 <= SOC <= 1/1
  0 <= SOC <= 1/1 -> ess_soc/1
  (sec->hrs)/1 -> 1\ess.plant.init.cap/1

== system AeroPropRefFranc/Propulsion and Aerodynamic Forces and Moments/S-Function/Battery Model/ess (battery)/plant/ess_plant_pngv_map_anl_PI_cstr/ess_cell/voltage calculation ==
  absolute SOC : Inport
  ess_cell_curr : Inport  Port=2
  ess_cell_curr_pol1 : Inport  Port=3
  ess_cell_curr_plo2 : Inport  Port=4
  Ohmic resist : Lookup  InputValues=ess.plant.init.rint.idx1_soc  Table=ess.plant.init.rint.map
  "Polarization resist 2 " : Lookup  InputValues=ess.plant.init.rpol2.idx1_soc  Table=ess.plant.init.rpol2.map
  Polarization resist2 : Lookup  InputValues=ess.plant.init.rpol1.idx1_soc  Table=ess.plant.init.rpol1.map
  Product1 : Product  InputSameDT=on  SaturateOnIntegerOverflow=on  OutDataTypeStr=Inherit: Same as first input
  Product2 : Product  InputSameDT=on  SaturateOnIntegerOverflow=on  OutDataTypeStr=Inherit: Same as first input
  Product3 : Product  InputSameDT=on  SaturateOnIntegerOverflow=on  OutDataTypeStr=Inherit: Same as first input
  Saturation : Saturate  UpperLimit=inf  LowerLimit=ess.plant.init.volt_min_burst
  Sum2 : Sum  Inputs=+---  InputSameDT=on  SaturateOnIntegerOverflow=on  OutDataTypeStr=Inherit: Same as first input
  Voc : Lookup  InputValues=ess.plant.init.voc.idx1_soc  Table=ess.plant.init.voc.map
  ess_cell_volt : Outport
  ess_cell_voc : Outport  Port=2
  ess_cell_rint : Outport  Port=3
  ess_cell_rpol1 : Outport  Port=4
  ess_cell_rpol2 : Outport  Port=5
  wires:
  Sum2/1 -> Saturation/1
  Ohmic resist/1 -> Product1/2, ess_cell_rint/1  "ess_rint_simu"
  ess_cell_curr/1 -> Product1/1
  Voc/1 -> Sum2/1, ess_cell_voc/1  "ess_voc_simu"
  absolute SOC/1 -> Voc/1, Ohmic resist/1, "Polarization resist 2 "/1, Polarization resist2/1
  Product1/1 -> Sum2/2
  ess_cell_curr_pol1/1 -> Product2/1
  Polarization resist2/1 -> Product2/2, ess_cell_rpol1/1  "ess_rpol1_simu"
  Product2/1 -> Sum2/3
  Product3/1 -> Sum2/4
  ess_cell_curr_plo2/1 -> Product3/1
  "Polarization resist 2 "/1 -> Product3/2, ess_cell_rpol2/1  "ess_rpol2_simu"
  Saturation/1 -> ess_cell_volt/1

== system AeroPropRefFranc/Propulsion and Aerodynamic Forces and Moments/S-Function/Battery Model/powerplant/ess (battery)/ctrl/ess_ctrl_pngv_map_anl_PI_cstr/PI controller for maximal charge power and current1 ==
  ess voltage : Inport
  ess curr : Inport  Port=2
  SOC : Inport  Port=3
  Burst maximal power : Lookup  InputValues=ess.plant.init.pwr_chg_10sec.idx1_soc  Table=ess.plant.init.pwr_chg_10sec.map  SaturateOnIntegerOverflow=off
  Continuous maximal power : Lookup  InputValues=ess.plant.init.pwr_chg.idx1_soc  Table=ess.plant.init.pwr_chg.map  SaturateOnIntegerOverflow=off
  Interpolation (curr) : Fcn  Expr=u(3)*u(1) + u(2)*(1-u(1))
  Interpolation (curr)1 : Fcn  Expr=u(3)*u(1) + u(2)*(1-u(1))
  Mux1 : Mux  Inputs=3
  Mux2 : Mux  Inputs=3
  "PI Ratio Calculator (curr) " : Subsystem
  PI Ratio Calculator (curr) 1 : Subsystem
  Product : Product  RndMeth=Zero
  Saturation : Saturate  UpperLimit=0  LowerLimit=-inf
  Saturation1 : Saturate  UpperLimit=0  LowerLimit=-inf
  "ess curr " : InportShadow  Port=2
  ess maximum current (burst charge) : Lookup  InputValues=ess.plant.init.curr_chg_burst_max.idx1_soc  Table=ess.plant.init.curr_chg_burst_max.map  SaturateOnIntegerOverflow=off
  ess maximum current (continuous charge) : Lookup  InputValues=ess.plant.init.curr_chg_cont_max.idx1_soc  Table=ess.plant.init.curr_chg_cont_max.map  SaturateOnIntegerOverflow=off
  ess.init.num_cell1 : Gain  Gain=ess.plant.init.num_cell  SaturateOnIntegerOverflow=on  OutDataTypeStr=Inherit: Same as input  ParamDataTypeStr=Inherit: Same as input
  ess.init.num_cell2 : Gain  Gain=ess.plant.init.num_cell  SaturateOnIntegerOverflow=on  OutDataTypeStr=Inherit: Same as input  ParamDataTypeStr=Inherit: Same as input
  ess.init.num_module_parallel1 : Gain  Gain=ess.plant.init.num_module_parallel
  ess.init.num_module_parallel5 : Gain  Gain=ess.plant.init.num_module_parallel
  Pwr_max_reg : Outport
  Curr_max_reg : Outport  Port=2
  wires:
  Saturation/1 -> "PI Ratio Calculator (curr) "/1(ess curr)
  "PI Ratio Calculator (curr) "/1(Current ratio) -> Mux1/1
  ess maximum current (burst charge)/1 -> ess.init.num_module_parallel1/1
  ess maximum current (continuous charge)/1 -> ess.init.num_module_parallel5/1
  ess curr/1 -> Saturation/1
  Mux1/1 -> Interpolation (curr)/1
  Interpolation (curr)/1 -> Curr_max_reg/1
  SOC/1 -> Continuous maximal power/1, Burst maximal power/1, ess maximum current (continuous charge)/1, ess maximum current (burst charge)/1
  Saturation1/1 -> PI Ratio Calculator (curr) 1/1(ess pwr)
  Continuous maximal power/1 -> ess.init.num_cell2/1
  Interpolation (curr)1/1 -> Pwr_max_reg/1
  Mux2/1 -> Interpolation (curr)1/1
  PI Ratio Calculator (curr) 1/1(pwr ratio) -> Mux2/1
  Burst maximal power/1 -> ess.init.num_cell1/1
  "ess curr "/1 -> Product/2
  ess voltage/1 -> Product/1
  Product/1 -> Saturation1/1
  ess.init.num_cell2/1 -> Mux2/2, PI Ratio Calculator (curr) 1/2(pwr max cont)
  ess.init.num_cell1/1 -> Mux2/3
  ess.init.num_module_parallel5/1 -> Mux1/2, "PI Ratio Calculator (curr) "/2(curr max cont)
  ess.init.num_module_parallel1/1 -> Mux1/3

== system AeroPropRefFranc/Propulsion and Aerodynamic Forces and Moments/S-Function/Battery Model/powerplant/ess (battery)/ctrl/ess_ctrl_pngv_map_anl_PI_cstr/PI controller for maximal discharge power and current1 ==
  ess voltage : Inport
  ess curr : Inport  Port=2
  SOC : Inport  Port=3
  Burst maximal power : Lookup  InputValues=ess.plant.init.pwr_dis_10sec.idx1_soc  Table=ess.plant.init.pwr_dis_10sec.map  SaturateOnIntegerOverflow=off
  Continuous maximal power : Lookup  InputValues=ess.plant.init.pwr_dis.idx1_soc  Table=ess.plant.init.pwr_dis.map  SaturateOnIntegerOverflow=off
  Interpolation (curr) : Fcn  Expr=u(3)*u(1) + u(2)*(1-u(1))
  Interpolation (curr)1 : Fcn  Expr=u(3)*u(1) + u(2)*(1-u(1))
  Mux1 : Mux  Inputs=3
  Mux2 : Mux  Inputs=3
  "PI Ratio Calculator (curr) " : Subsystem
  PI Ratio Calculator (curr) 1 : Subsystem
  Product : Product  RndMeth=Zero
  Saturation : Saturate  UpperLimit=inf  LowerLimit=0
  Saturation1 : Saturate  UpperLimit=inf  LowerLimit=0
  "ess curr " : InportShadow  Port=2
  ess maximum current (burst discharge)1 : Lookup  InputValues=ess.plant.init.curr_dis_burst_max.idx1_soc  Table=ess.plant.init.curr_dis_burst_max.map  SaturateOnIntegerOverflow=off
  "ess maximum current (continuous discharge) " : Lookup  InputValues=ess.plant.init.curr_dis_cont_max.idx1_soc  Table=ess.plant.init.curr_dis_cont_max.map  SaturateOnIntegerOverflow=off
  ess.init.num_cell1 : Gain  Gain=ess.plant.init.num_cell  SaturateOnIntegerOverflow=on  OutDataTypeStr=Inherit: Same as input  ParamDataTypeStr=Inherit: Same as input
  ess.init.num_cell2 : Gain  Gain=ess.plant.init.num_cell  SaturateOnIntegerOverflow=on  OutDataTypeStr=Inherit: Same as input  ParamDataTypeStr=Inherit: Same as input
  ess.init.num_module_parallel1 : Gain  Gain=ess.plant.init.num_module_parallel
  ess.init.num_module_parallel5 : Gain  Gain=ess.plant.init.num_module_parallel
  Curr_max_prop : Outport
  Pwr_max_prop : Outport  Port=2
  wires:
  Interpolation (curr)/1 -> Curr_max_prop/1
  Mux1/1 -> Interpolation (curr)/1
  ess curr/1 -> Saturation/1
  "ess maximum current (continuous discharge) "/1 -> ess.init.num_module_parallel5/1
  ess maximum current (burst discharge)1/1 -> ess.init.num_module_parallel1/1
  "PI Ratio Calculator (curr) "/1(Current ratio) -> Mux1/1
  Saturation/1 -> "PI Ratio Calculator (curr) "/1(ess curr)
  SOC/1 -> Continuous maximal power/1, Burst maximal power/1, "ess maximum current (continuous discharge) "/1, ess maximum current (burst discharge)1/1
  Saturation1/1 -> PI Ratio Calculator (curr) 1/1(ess pwr)
  Continuous maximal power/1 -> ess.init.num_cell1/1
  Interpolation (curr)1/1 -> Pwr_max_prop/1
  Mux2/1 -> Interpolation (curr)1/1
  PI Ratio Calculator (curr) 1/1(pwr ratio) -> Mux2/1
  Burst maximal power/1 -> ess.init.num_cell2/1
  "ess curr "/1 -> Product/2
  ess voltage/1 -> Product/1
  Product/1 -> Saturation1/1
  ess.init.num_cell1/1 -> Mux2/2, PI Ratio Calculator (curr) 1/2(pwr max cont)
  ess.init.num_cell2/1 -> Mux2/3
  ess.init.num_module_parallel5/1 -> "PI Ratio Calculator (curr) "/2(curr max cont), Mux1/2
  ess.init.num_module_parallel1/1 -> Mux1/3
